simulink model "testbench_2"  (R2022b)
settings: Solver=VariableStepAuto  StartTime=0.0  StopTime=3600  RelTol=1e-3
undefined symbols (not defined in the file): battery_builder_rtmsupport, gcbh
libraries: nesl_utility x10, GD_Batterymodel_lib x8, fl_lib x2, BatteryCurrentManagement x1, BatteryBalancing x1
(part 2 of 2)

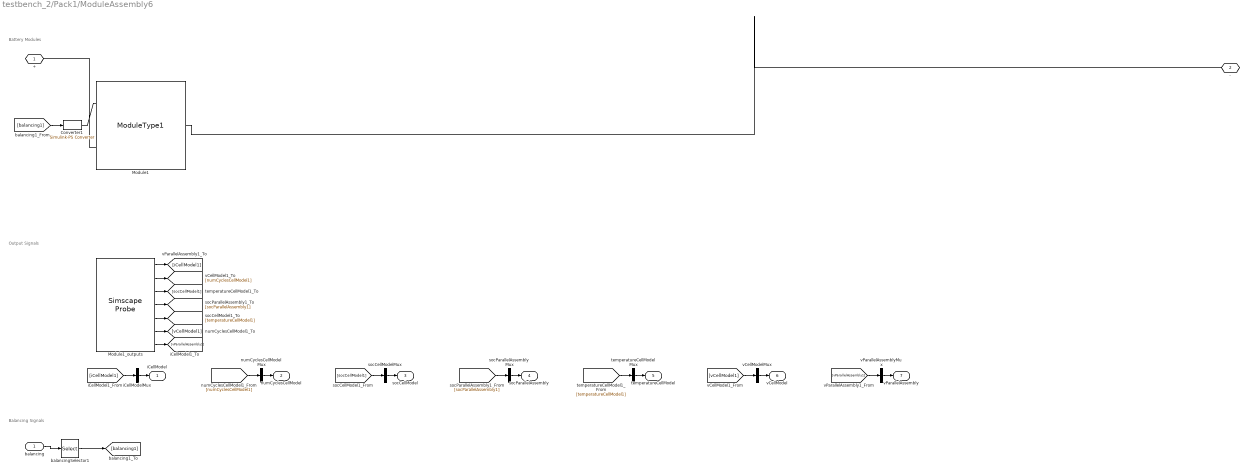
== system testbench_2/Pack1/ModuleAssembly6 ==
  note: Battery Modules
  note: Output Signals
  note: Balancing Signals
  balancing : Inport  PortDimensions=14
  Converter1 : nesl_utility/Simulink-PS Converter  PhysicalDomain=network_engine_domain  SubClassName=ps_input  LeftPortType=input  RightPortType=output  PseudoPeriodic=off  Frequencies=[]  NoiseDistribution=none  NoiseParameters=[]  Unit=1  AffineConversion=off  FilteringAndDerivatives=provide  SimscapeFilterOrder=1  InputFilterTimeConstant=0.001  UdotUserProvided=0
  Module1 : GD_Batterymodel_lib/Modules/ModuleType1  SOC_vec=[0, .1, .25, .5, .75, .9, 1]  T_vec=[278, 293, 313] K  V0_mat=[3.49, 3.5, 3.51; 3.55, 3.57, 3.56; 3.62, 3.63, 3.64; 3.71, 3.71, 3.72; 3.91, 3.93, 3.94; 4.07, 4.08, 4.08; 4.19, 4.19, 4.19] V  V_range=[0, inf] V  R0_mat=[.0117, .0085, .009; .011, .0085, .009; .0114, .0087, .0092; .0107, .0082, .0088; .0107, .0083, .0091; .0113, .0085, .0089; .0116, .0085, .0089] Ohm  AH=27 A*hr  extrapolation_option=simscape.enum.extrapolation.nearest  thermal_mass=100 J/K  CellBalancingClosedResistance=0.01 Ohm  CellBalancingOpenConductance=1e-8 1/Ohm  CellBalancingThreshold=0.5  CellBalancingResistance=50 Ohm  P=3  S=14  iCellModel_specify=off  iCellModel_priority=None  iCellModel=repmat(0, 42, 1) A  iCellModel_nominal_specify=off  iCellModel_nominal_unit=A  iCellModel_nominal_value=1  vCellModel_specify=off  vCellModel_priority=None  vCellModel=repmat(0, 42, 1) V  vCellModel_nominal_specify=off  vCellModel_nominal_unit=V  vCellModel_nominal_value=1  socCellModel_specify=off  socCellModel_priority=High  socCellModel=repmat(1, 42, 1)  socCellModel_nominal_specify=off  socCellModel_nominal_unit=1  socCellModel_nominal_value=1  numCyclesCellModel_specify=off  numCyclesCellModel_priority=High  numCyclesCellModel=repmat(0, 42, 1)  numCyclesCellModel_nominal_specify=off  numCyclesCellModel_nominal_unit=1  numCyclesCellModel_nominal_value=1  temperatureCellModel_specify=off  temperatureCellModel_priority=High  temperatureCellModel=repmat(298.15, 42, 1) K  temperatureCellModel_nominal_specify=off  temperatureCellModel_nominal_unit=K  temperatureCellModel_nominal_value=1  vParallelAssembly_specify=off  vParallelAssembly_priority=None  vParallelAssembly=repmat(0, 14, 1) V  vParallelAssembly_nominal_specify=off  vParallelAssembly_nominal_unit=V  vParallelAssembly_nominal_value=1  socParallelAssembly_specify=off  socParallelAssembly_priority=None  socParallelAssembly=repmat(1, 14, 1)  socParallelAssembly_nominal_specify=off  socParallelAssembly_nominal_unit=1  socParallelAssembly_nominal_value=1
      settings: InternalSimscapePortConfiguration="{\"Bottom\":[{\"id\":\"n\",\"label\":\"-\",\"type\":\"foundation.electrical.electrical\"}],\"Left\":[{\"id\":\"enableCellBalancing\",\"label\":\"CB\",\"type\":\"input\"}],\"Right\":[],\"Top\":[{\"id\":\"p\",\"label\":\"+\",\"type\":\"foundation.electrical.electrical\"}]}"
  Module1_outputs : SimscapeProbe  BoundBlock=727  Variables={iCellModel, numCyclesCellModel, socCellModel, socParallelAssembly, temperatureCellModel, vCellModel, vParallelAssembly}
  balancingSelector1 : Selector  InputPortWidth=14  IndexOptions=Index vector (dialog)  Indices="[1   2   3   4   5   6   7   8   9  10  11  12  13  14]"  OutputSizes=1
  iCellModelMux : Mux  Inputs=1
  numCyclesCellModelMux : Mux  Inputs=1
  socCellModelMux : Mux  Inputs=1
  socParallelAssemblyMux : Mux  Inputs=1
  temperatureCellModelMux : Mux  Inputs=1
  vCellModelMux : Mux  Inputs=1
  vParallelAssemblyMux : Mux  Inputs=1
  + : PMIOPort  Side=Left
  - : PMIOPort  Port=2  Side=Right
  iCellModel : Outport
  numCyclesCellModel : Outport  Port=2
  socCellModel : Outport  Port=3
  socParallelAssembly : Outport  Port=4
  temperatureCellModel : Outport  Port=5
  vCellModel : Outport  Port=6
  vParallelAssembly : Outport  Port=7
  wires:
  Module1_outputs/7 -> [vParallelAssembly1]
  iCellModelMux/1 -> iCellModel/1
  [iCellModel1] -> iCellModelMux/1
  Module1_outputs/6 -> [vCellModel1]
  numCyclesCellModelMux/1 -> numCyclesCellModel/1
  [numCyclesCellModel1] -> numCyclesCellModelMux/1
  Module1_outputs/5 -> [temperatureCellModel1]
  socCellModelMux/1 -> socCellModel/1
  [socCellModel1] -> socCellModelMux/1
  Module1_outputs/4 -> [socParallelAssembly1]
  socParallelAssemblyMux/1 -> socParallelAssembly/1
  [socParallelAssembly1] -> socParallelAssemblyMux/1
  Module1_outputs/3 -> [socCellModel1]
  temperatureCellModelMux/1 -> temperatureCellModel/1
  [temperatureCellModel1] -> temperatureCellModelMux/1
  Module1_outputs/2 -> [numCyclesCellModel1]
  vCellModelMux/1 -> vCellModel/1
  [vCellModel1] -> vCellModelMux/1
  Module1_outputs/1 -> [iCellModel1]
  vParallelAssemblyMux/1 -> vParallelAssembly/1
  [vParallelAssembly1] -> vParallelAssemblyMux/1
  balancing/1 -> balancingSelector1/1
  balancingSelector1/1 -> [balancing1]
  [balancing1] -> Converter1/1
  connections:
  Module1/LConn2 -- +/RConn1
  Module1/RConn1 -- -/RConn1
  Converter1/RConn1 -- Module1/LConn1

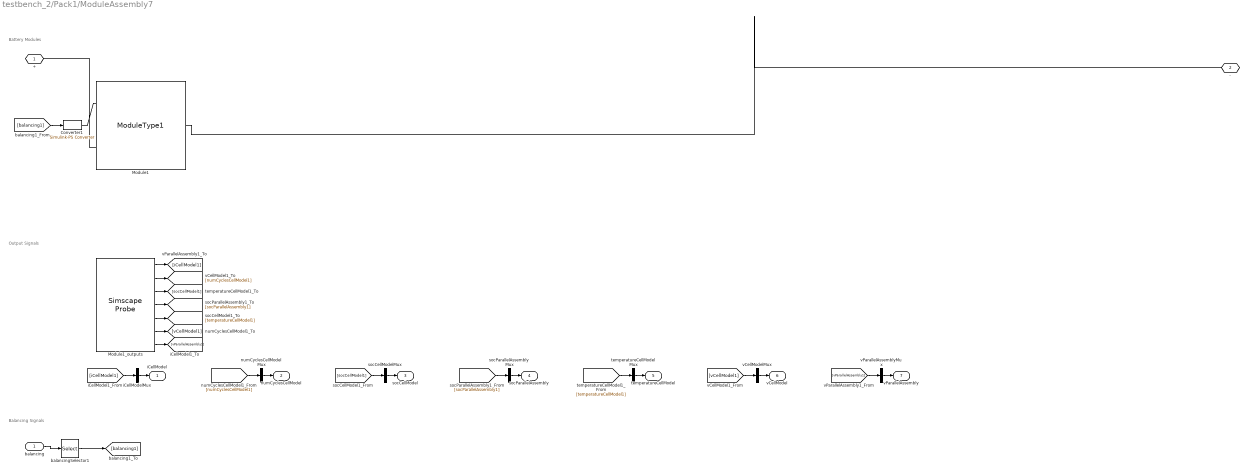
== system testbench_2/Pack1/ModuleAssembly7 ==
  note: Battery Modules
  note: Output Signals
  note: Balancing Signals
  balancing : Inport  PortDimensions=14
  Converter1 : nesl_utility/Simulink-PS Converter  PhysicalDomain=network_engine_domain  SubClassName=ps_input  LeftPortType=input  RightPortType=output  PseudoPeriodic=off  Frequencies=[]  NoiseDistribution=none  NoiseParameters=[]  Unit=1  AffineConversion=off  FilteringAndDerivatives=provide  SimscapeFilterOrder=1  InputFilterTimeConstant=0.001  UdotUserProvided=0
  Module1 : GD_Batterymodel_lib/Modules/ModuleType1  SOC_vec=[0, .1, .25, .5, .75, .9, 1]  T_vec=[278, 293, 313] K  V0_mat=[3.49, 3.5, 3.51; 3.55, 3.57, 3.56; 3.62, 3.63, 3.64; 3.71, 3.71, 3.72; 3.91, 3.93, 3.94; 4.07, 4.08, 4.08; 4.19, 4.19, 4.19] V  V_range=[0, inf] V  R0_mat=[.0117, .0085, .009; .011, .0085, .009; .0114, .0087, .0092; .0107, .0082, .0088; .0107, .0083, .0091; .0113, .0085, .0089; .0116, .0085, .0089] Ohm  AH=27 A*hr  extrapolation_option=simscape.enum.extrapolation.nearest  thermal_mass=100 J/K  CellBalancingClosedResistance=0.01 Ohm  CellBalancingOpenConductance=1e-8 1/Ohm  CellBalancingThreshold=0.5  CellBalancingResistance=50 Ohm  P=3  S=14  iCellModel_specify=off  iCellModel_priority=None  iCellModel=repmat(0, 42, 1) A  iCellModel_nominal_specify=off  iCellModel_nominal_unit=A  iCellModel_nominal_value=1  vCellModel_specify=off  vCellModel_priority=None  vCellModel=repmat(0, 42, 1) V  vCellModel_nominal_specify=off  vCellModel_nominal_unit=V  vCellModel_nominal_value=1  socCellModel_specify=off  socCellModel_priority=High  socCellModel=repmat(1, 42, 1)  socCellModel_nominal_specify=off  socCellModel_nominal_unit=1  socCellModel_nominal_value=1  numCyclesCellModel_specify=off  numCyclesCellModel_priority=High  numCyclesCellModel=repmat(0, 42, 1)  numCyclesCellModel_nominal_specify=off  numCyclesCellModel_nominal_unit=1  numCyclesCellModel_nominal_value=1  temperatureCellModel_specify=off  temperatureCellModel_priority=High  temperatureCellModel=repmat(298.15, 42, 1) K  temperatureCellModel_nominal_specify=off  temperatureCellModel_nominal_unit=K  temperatureCellModel_nominal_value=1  vParallelAssembly_specify=off  vParallelAssembly_priority=None  vParallelAssembly=repmat(0, 14, 1) V  vParallelAssembly_nominal_specify=off  vParallelAssembly_nominal_unit=V  vParallelAssembly_nominal_value=1  socParallelAssembly_specify=off  socParallelAssembly_priority=None  socParallelAssembly=repmat(1, 14, 1)  socParallelAssembly_nominal_specify=off  socParallelAssembly_nominal_unit=1  socParallelAssembly_nominal_value=1
      settings: InternalSimscapePortConfiguration="{\"Bottom\":[{\"id\":\"n\",\"label\":\"-\",\"type\":\"foundation.electrical.electrical\"}],\"Left\":[{\"id\":\"enableCellBalancing\",\"label\":\"CB\",\"type\":\"input\"}],\"Right\":[],\"Top\":[{\"id\":\"p\",\"label\":\"+\",\"type\":\"foundation.electrical.electrical\"}]}"
  Module1_outputs : SimscapeProbe  BoundBlock=768  Variables={iCellModel, numCyclesCellModel, socCellModel, socParallelAssembly, temperatureCellModel, vCellModel, vParallelAssembly}
  balancingSelector1 : Selector  InputPortWidth=14  IndexOptions=Index vector (dialog)  Indices="[1   2   3   4   5   6   7   8   9  10  11  12  13  14]"  OutputSizes=1
  iCellModelMux : Mux  Inputs=1
  numCyclesCellModelMux : Mux  Inputs=1
  socCellModelMux : Mux  Inputs=1
  socParallelAssemblyMux : Mux  Inputs=1
  temperatureCellModelMux : Mux  Inputs=1
  vCellModelMux : Mux  Inputs=1
  vParallelAssemblyMux : Mux  Inputs=1
  + : PMIOPort  Side=Left
  - : PMIOPort  Port=2  Side=Right
  iCellModel : Outport
  numCyclesCellModel : Outport  Port=2
  socCellModel : Outport  Port=3
  socParallelAssembly : Outport  Port=4
  temperatureCellModel : Outport  Port=5
  vCellModel : Outport  Port=6
  vParallelAssembly : Outport  Port=7
  wires:
  Module1_outputs/7 -> [vParallelAssembly1]
  iCellModelMux/1 -> iCellModel/1
  [iCellModel1] -> iCellModelMux/1
  Module1_outputs/6 -> [vCellModel1]
  numCyclesCellModelMux/1 -> numCyclesCellModel/1
  [numCyclesCellModel1] -> numCyclesCellModelMux/1
  Module1_outputs/5 -> [temperatureCellModel1]
  socCellModelMux/1 -> socCellModel/1
  [socCellModel1] -> socCellModelMux/1
  Module1_outputs/4 -> [socParallelAssembly1]
  socParallelAssemblyMux/1 -> socParallelAssembly/1
  [socParallelAssembly1] -> socParallelAssemblyMux/1
  Module1_outputs/3 -> [socCellModel1]
  temperatureCellModelMux/1 -> temperatureCellModel/1
  [temperatureCellModel1] -> temperatureCellModelMux/1
  Module1_outputs/2 -> [numCyclesCellModel1]
  vCellModelMux/1 -> vCellModel/1
  [vCellModel1] -> vCellModelMux/1
  Module1_outputs/1 -> [iCellModel1]
  vParallelAssemblyMux/1 -> vParallelAssembly/1
  [vParallelAssembly1] -> vParallelAssemblyMux/1
  balancing/1 -> balancingSelector1/1
  balancingSelector1/1 -> [balancing1]
  [balancing1] -> Converter1/1
  connections:
  Module1/LConn2 -- +/RConn1
  Module1/RConn1 -- -/RConn1
  Converter1/RConn1 -- Module1/LConn1

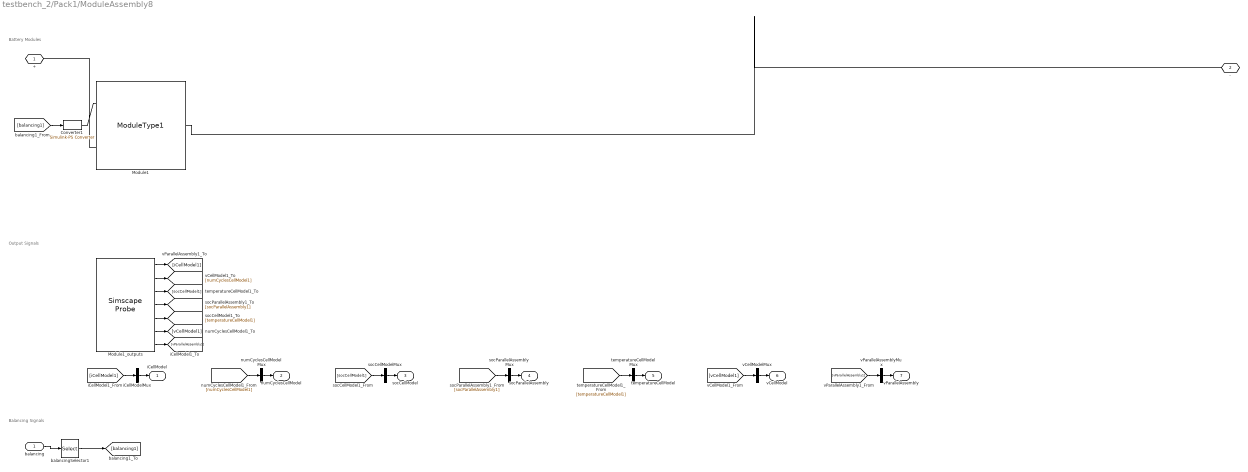
== system testbench_2/Pack1/ModuleAssembly8 ==
  note: Battery Modules
  note: Output Signals
  note: Balancing Signals
  balancing : Inport  PortDimensions=14
  Converter1 : nesl_utility/Simulink-PS Converter  PhysicalDomain=network_engine_domain  SubClassName=ps_input  LeftPortType=input  RightPortType=output  PseudoPeriodic=off  Frequencies=[]  NoiseDistribution=none  NoiseParameters=[]  Unit=1  AffineConversion=off  FilteringAndDerivatives=provide  SimscapeFilterOrder=1  InputFilterTimeConstant=0.001  UdotUserProvided=0
  Module1 : GD_Batterymodel_lib/Modules/ModuleType1  SOC_vec=[0, .1, .25, .5, .75, .9, 1]  T_vec=[278, 293, 313] K  V0_mat=[3.49, 3.5, 3.51; 3.55, 3.57, 3.56; 3.62, 3.63, 3.64; 3.71, 3.71, 3.72; 3.91, 3.93, 3.94; 4.07, 4.08, 4.08; 4.19, 4.19, 4.19] V  V_range=[0, inf] V  R0_mat=[.0117, .0085, .009; .011, .0085, .009; .0114, .0087, .0092; .0107, .0082, .0088; .0107, .0083, .0091; .0113, .0085, .0089; .0116, .0085, .0089] Ohm  AH=27 A*hr  extrapolation_option=simscape.enum.extrapolation.nearest  thermal_mass=100 J/K  CellBalancingClosedResistance=0.01 Ohm  CellBalancingOpenConductance=1e-8 1/Ohm  CellBalancingThreshold=0.5  CellBalancingResistance=50 Ohm  P=3  S=14  iCellModel_specify=off  iCellModel_priority=None  iCellModel=repmat(0, 42, 1) A  iCellModel_nominal_specify=off  iCellModel_nominal_unit=A  iCellModel_nominal_value=1  vCellModel_specify=off  vCellModel_priority=None  vCellModel=repmat(0, 42, 1) V  vCellModel_nominal_specify=off  vCellModel_nominal_unit=V  vCellModel_nominal_value=1  socCellModel_specify=off  socCellModel_priority=High  socCellModel=repmat(1, 42, 1)  socCellModel_nominal_specify=off  socCellModel_nominal_unit=1  socCellModel_nominal_value=1  numCyclesCellModel_specify=off  numCyclesCellModel_priority=High  numCyclesCellModel=repmat(0, 42, 1)  numCyclesCellModel_nominal_specify=off  numCyclesCellModel_nominal_unit=1  numCyclesCellModel_nominal_value=1  temperatureCellModel_specify=off  temperatureCellModel_priority=High  temperatureCellModel=repmat(298.15, 42, 1) K  temperatureCellModel_nominal_specify=off  temperatureCellModel_nominal_unit=K  temperatureCellModel_nominal_value=1  vParallelAssembly_specify=off  vParallelAssembly_priority=None  vParallelAssembly=repmat(0, 14, 1) V  vParallelAssembly_nominal_specify=off  vParallelAssembly_nominal_unit=V  vParallelAssembly_nominal_value=1  socParallelAssembly_specify=off  socParallelAssembly_priority=None  socParallelAssembly=repmat(1, 14, 1)  socParallelAssembly_nominal_specify=off  socParallelAssembly_nominal_unit=1  socParallelAssembly_nominal_value=1
      settings: InternalSimscapePortConfiguration="{\"Bottom\":[{\"id\":\"n\",\"label\":\"-\",\"type\":\"foundation.electrical.electrical\"}],\"Left\":[{\"id\":\"enableCellBalancing\",\"label\":\"CB\",\"type\":\"input\"}],\"Right\":[],\"Top\":[{\"id\":\"p\",\"label\":\"+\",\"type\":\"foundation.electrical.electrical\"}]}"
  Module1_outputs : SimscapeProbe  BoundBlock=809  Variables={iCellModel, numCyclesCellModel, socCellModel, socParallelAssembly, temperatureCellModel, vCellModel, vParallelAssembly}
  balancingSelector1 : Selector  InputPortWidth=14  IndexOptions=Index vector (dialog)  Indices="[1   2   3   4   5   6   7   8   9  10  11  12  13  14]"  OutputSizes=1
  iCellModelMux : Mux  Inputs=1
  numCyclesCellModelMux : Mux  Inputs=1
  socCellModelMux : Mux  Inputs=1
  socParallelAssemblyMux : Mux  Inputs=1
  temperatureCellModelMux : Mux  Inputs=1
  vCellModelMux : Mux  Inputs=1
  vParallelAssemblyMux : Mux  Inputs=1
  + : PMIOPort  Side=Left
  - : PMIOPort  Port=2  Side=Right
  iCellModel : Outport
  numCyclesCellModel : Outport  Port=2
  socCellModel : Outport  Port=3
  socParallelAssembly : Outport  Port=4
  temperatureCellModel : Outport  Port=5
  vCellModel : Outport  Port=6
  vParallelAssembly : Outport  Port=7
  wires:
  Module1_outputs/7 -> [vParallelAssembly1]
  iCellModelMux/1 -> iCellModel/1
  [iCellModel1] -> iCellModelMux/1
  Module1_outputs/6 -> [vCellModel1]
  numCyclesCellModelMux/1 -> numCyclesCellModel/1
  [numCyclesCellModel1] -> numCyclesCellModelMux/1
  Module1_outputs/5 -> [temperatureCellModel1]
  socCellModelMux/1 -> socCellModel/1
  [socCellModel1] -> socCellModelMux/1
  Module1_outputs/4 -> [socParallelAssembly1]
  socParallelAssemblyMux/1 -> socParallelAssembly/1
  [socParallelAssembly1] -> socParallelAssemblyMux/1
  Module1_outputs/3 -> [socCellModel1]
  temperatureCellModelMux/1 -> temperatureCellModel/1
  [temperatureCellModel1] -> temperatureCellModelMux/1
  Module1_outputs/2 -> [numCyclesCellModel1]
  vCellModelMux/1 -> vCellModel/1
  [vCellModel1] -> vCellModelMux/1
  Module1_outputs/1 -> [iCellModel1]
  vParallelAssemblyMux/1 -> vParallelAssembly/1
  [vParallelAssembly1] -> vParallelAssemblyMux/1
  balancing/1 -> balancingSelector1/1
  balancingSelector1/1 -> [balancing1]
  [balancing1] -> Converter1/1
  connections:
  Module1/LConn2 -- +/RConn1
  Module1/RConn1 -- -/RConn1
  Converter1/RConn1 -- Module1/LConn1
